simulink model "steeringwheel_clean"  (Simulink 9.2)
settings: Solver=ode45  StartTime=0.0  StopTime=60  MaxStep=1e-3  RelTol=1e-6
settings Model: Creator=jinwooro  LastModifiedBy=jinwooro
settings DataIOCC: LimitDataPoints=off  SaveFormat=Dataset  SignalLoggingSaveFormat=Dataset
settings OptimizationCC: LifeSpan=auto
settings DebuggingCC: UnderspecifiedInitializationDetection=Simplified  MergeDetectMultiDrivingBlocksExec=error  FcnCallInpInsideContextMsg=error  StateNameClashWarn=none  SFUnexpectedBacktrackingDiag=error  SFNoUnconditionalDefaultTransitionDiag=error  SFExecutionAtInitializationDiag=warning
settings HardwareCC: ProdBitPerPointer=64  ProdBitPerSizeT=64  ProdBitPerPtrDiffT=64  ProdLargestAtomicFloat=Float  ProdIntDivRoundTo=Zero  ProdEndianess=LittleEndian  ProdWordSize=64  ProdHWDeviceType=Intel->x86-64 (Windows64)
settings ModelReferenceCC: PropagateSignalLabelsOutOfModel=on
settings SFSimCC: SimUseLocalCustomCode=on
settings RTWCC: RTWUseLocalCustomCode=on
settings CodeAppCC: StateflowObjectComments=off
settings GRTTargetCC: TargetLangStandard=C99 (ISO)  GeneratePreprocessorConditionals=Use local settings  CombineOutputUpdateFcns=on  GRTInterface=off
settings ConfigComp: CovMetricSettings=dwe  CovHtmlReporting=off  CovSaveCumulativeToWorkspaceVar=off  CovSaveSingleToWorkspaceVar=off  CovExternalEMLEnable=on

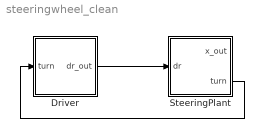
== system steeringwheel_clean ==
  Driver : Stateflow chart  TreatAsAtomicUnit=on
  SteeringPlant : Stateflow chart  TreatAsAtomicUnit=on
  wires:
  SteeringPlant/2(turn) -> Driver/1(turn)
  Driver/1(dr_out) -> SteeringPlant/1(dr)

== stateflow chart Driver ==
  settings: updateMethod=CONTINUOUS
  state ConstLeftTurn
    du:
    dr_out = 0.1;
  state ConstRightTurn
    du:
    dr_out = -4;
  (default) -> ConstLeftTurn
  ConstLeftTurn -> ConstRightTurn : [turn == 0]
  ConstRightTurn -> ConstLeftTurn : [turn == 1]
  data: dr_out output double; turn input double

== stateflow chart SteeringPlant ==
  settings: updateMethod=CONTINUOUS
  state SteeringLeft
    du:
    r_dot = dr;
    x_out = cos(r);
  state SteeringRight
    du:
    r_dot = dr;
    x_out = cos(r);
  (default) -> SteeringLeft : {r = 0.5 * pi;}
  SteeringLeft -> SteeringRight : [cos(r) <= -0.99]
      | {turn = 1;}
  SteeringRight -> SteeringLeft : [cos(r) >= 0.99]
      | {turn = 0;}
  data: r local double; x_out output double; dr input double; turn output double
  data r settings: updateMethod=SF_CONTINUOUS_TIME_DATA
